simulink model "Sillas_Rosario_TP02_Simulink"  (R2014a)
settings: Solver=ode45  StartTime=0.0  StopTime=7  RelTol=1e-3
libraries: simulink x3
settings Model: Creator=Silas  LastModifiedBy=Silas

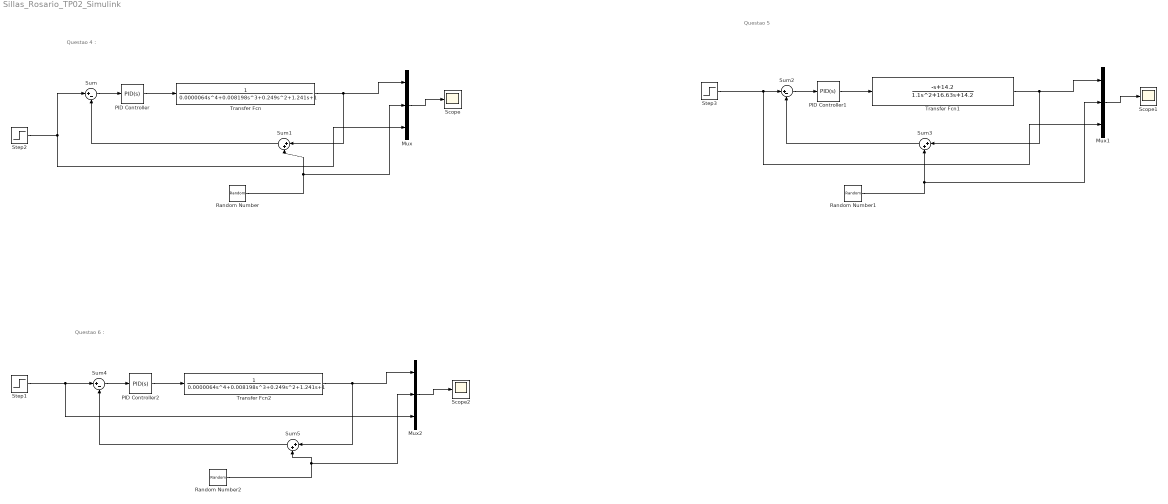
== system Sillas_Rosario_TP02_Simulink ==
  note: Questao 5
  note: Questao 4 :
  note: Questao 6 :
  Mux : Mux  Inputs=3
  Mux1 : Mux  Inputs=3
  Mux2 : Mux  Inputs=3
  PID Controller : simulink/Continuous/PID Controller  Controller=PID  TimeDomain=Continuous-time  SampleTime=1  IntegratorMethod=Forward Euler  FilterMethod=Forward Euler  Form=Parallel  P=4.9337  I=4.884363  D=0.80814  N=100  InitialConditionSource=internal  InitialConditionForIntegrator=0  InitialConditionForFilter=0  ExternalReset=none  LimitOutput=off  UpperSaturationLimit=inf  LowerSaturationLimit=-inf  LinearizeAsGain=on  AntiWindupMode=none  Kb=1  TrackingMode=off  Kt=1  PParamMin=[]  PParamMax=[]  IParamMin=[]  IParamMax=[]  DParamMin=[]  DParamMax=[]  NParamMin=[]  NParamMax=[]  KbParamMin=[]  KbParamMax=[]  KtParamMin=[]  KtParamMax=[]  POutMin=[]  POutMax=[]  IOutMin=[]  IOutMax=[]  DOutMin=[]  DOutMax=[]  NOutMin=[]  NOutMax=[]  KbOutMin=[]  KbOutMax=[]  KtOutMin=[]  KtOutMax=[]  IntegratorOutMin=[]  IntegratorOutMax=[]  FilterOutMin=[]  FilterOutMax=[]  SumOutMin=[]  SumOutMax=[]  SumI1OutMin=[]  SumI1OutMax=[]  SumI2OutMin=[]  SumI2OutMax=[]  SumI3OutMin=[]  SumI3OutMax=[]  SumDOutMin=[]  SumDOutMax=[]  SaturationOutMin=[]  SaturationOutMax=[]  IntegratorContinuousStateAttributes=''  IntegratorStateMustResolveToSignalObject=off  IntegratorRTWStateStorageClass=Auto  FilterContinuousStateAttributes=''  FilterStateMustResolveToSignalObject=off  FilterRTWStateStorageClass=Auto
  PID Controller1 : simulink/Continuous/PID Controller  Controller=PID  TimeDomain=Continuous-time  SampleTime=1  IntegratorMethod=Forward Euler  FilterMethod=Forward Euler  Form=Parallel  P=3.42561  I=3.5286  D=0  N=100  InitialConditionSource=internal  InitialConditionForIntegrator=0  InitialConditionForFilter=0  ExternalReset=none  LimitOutput=off  UpperSaturationLimit=inf  LowerSaturationLimit=-inf  LinearizeAsGain=on  AntiWindupMode=none  Kb=1  TrackingMode=off  Kt=1  PParamMin=[]  PParamMax=[]  IParamMin=[]  IParamMax=[]  DParamMin=[]  DParamMax=[]  NParamMin=[]  NParamMax=[]  KbParamMin=[]  KbParamMax=[]  KtParamMin=[]  KtParamMax=[]  POutMin=[]  POutMax=[]  IOutMin=[]  IOutMax=[]  DOutMin=[]  DOutMax=[]  NOutMin=[]  NOutMax=[]  KbOutMin=[]  KbOutMax=[]  KtOutMin=[]  KtOutMax=[]  IntegratorOutMin=[]  IntegratorOutMax=[]  FilterOutMin=[]  FilterOutMax=[]  SumOutMin=[]  SumOutMax=[]  SumI1OutMin=[]  SumI1OutMax=[]  SumI2OutMin=[]  SumI2OutMax=[]  SumI3OutMin=[]  SumI3OutMax=[]  SumDOutMin=[]  SumDOutMax=[]  SaturationOutMin=[]  SaturationOutMax=[]  IntegratorContinuousStateAttributes=''  IntegratorStateMustResolveToSignalObject=off  IntegratorRTWStateStorageClass=Auto  FilterContinuousStateAttributes=''  FilterStateMustResolveToSignalObject=off  FilterRTWStateStorageClass=Auto
  PID Controller2 : simulink/Continuous/PID Controller  Controller=PID  TimeDomain=Continuous-time  SampleTime=1  IntegratorMethod=Forward Euler  FilterMethod=Forward Euler  Form=Parallel  P=3.42561  I=3.5286  D=0  N=100  InitialConditionSource=internal  InitialConditionForIntegrator=0  InitialConditionForFilter=0  ExternalReset=none  LimitOutput=off  UpperSaturationLimit=inf  LowerSaturationLimit=-inf  LinearizeAsGain=on  AntiWindupMode=none  Kb=1  TrackingMode=off  Kt=1  PParamMin=[]  PParamMax=[]  IParamMin=[]  IParamMax=[]  DParamMin=[]  DParamMax=[]  NParamMin=[]  NParamMax=[]  KbParamMin=[]  KbParamMax=[]  KtParamMin=[]  KtParamMax=[]  POutMin=[]  POutMax=[]  IOutMin=[]  IOutMax=[]  DOutMin=[]  DOutMax=[]  NOutMin=[]  NOutMax=[]  KbOutMin=[]  KbOutMax=[]  KtOutMin=[]  KtOutMax=[]  IntegratorOutMin=[]  IntegratorOutMax=[]  FilterOutMin=[]  FilterOutMax=[]  SumOutMin=[]  SumOutMax=[]  SumI1OutMin=[]  SumI1OutMax=[]  SumI2OutMin=[]  SumI2OutMax=[]  SumI3OutMin=[]  SumI3OutMax=[]  SumDOutMin=[]  SumDOutMax=[]  SaturationOutMin=[]  SaturationOutMax=[]  IntegratorContinuousStateAttributes=''  IntegratorStateMustResolveToSignalObject=off  IntegratorRTWStateStorageClass=Auto  FilterContinuousStateAttributes=''  FilterStateMustResolveToSignalObject=off  FilterRTWStateStorageClass=Auto
  Random Number : RandomNumber  Variance=0.01  SampleTime=0.01
  Random Number1 : RandomNumber  Variance=0.001  SampleTime=0.01
  Random Number2 : RandomNumber  Variance=0.001  SampleTime=0.01
  Scope : Scope
      settings: TimeRange=3.5  YMin=-0.5  YMax=2.5
  Scope1 : Scope
      settings: TimeRange=3.5  YMin=-0.5  YMax=2.5
  Scope2 : Scope
      settings: TimeRange=3.5  YMin=-0.5  YMax=2.5  SaveName=ScopeData2
  Step1 : Step  Time=4  Before=1  After=3  SampleTime=0
  Step2 : Step  Time=4  Before=1  After=2  SampleTime=0
  Step3 : Step  Time=4  Before=1  After=3  SampleTime=0
  Sum : Sum  Inputs=|+-
  Sum1 : Sum  Inputs=|++
  Sum2 : Sum  Inputs=|+-
  Sum3 : Sum  Inputs=|++
  Sum4 : Sum  Inputs=|+-
  Sum5 : Sum  Inputs=|++
  Transfer Fcn : TransferFcn  Denominator=[0.0000064 0.008198 0.249 1.241 1]
  Transfer Fcn1 : TransferFcn  Numerator=[-1 14.2]  Denominator=[1.1 16.63 14.2]
  Transfer Fcn2 : TransferFcn  Denominator=[0.0000064 0.008198 0.249 1.241 1]
  wires:
  Sum/1 -> PID Controller/1
  Transfer Fcn/1 -> Mux/1, Sum1/1
  Sum1/1 -> Sum/2
  Mux/1 -> Scope/1
  Step2/1 -> Sum/1, Mux/3
  Random Number/1 -> Mux/2, Sum1/2
  PID Controller/1 -> Transfer Fcn/1
  Sum2/1 -> PID Controller1/1
  Transfer Fcn1/1 -> Sum3/1, Mux1/1
  Sum3/1 -> Sum2/2
  Mux1/1 -> Scope1/1
  Step3/1 -> Mux1/3, Sum2/1
  Random Number1/1 -> Mux1/2, Sum3/2
  PID Controller1/1 -> Transfer Fcn1/1
  Sum4/1 -> PID Controller2/1
  Transfer Fcn2/1 -> Mux2/1, Sum5/1
  Sum5/1 -> Sum4/2
  Mux2/1 -> Scope2/1
  Random Number2/1 -> Mux2/2, Sum5/2
  PID Controller2/1 -> Transfer Fcn2/1
  Step1/1 -> Mux2/3, Sum4/1
